simulink model "brake_ctrl"  (R2025b)
settings: Solver=VariableStepAuto  StartTime=0.0  StopTime=10.0  RelTol=1e-3
settings Model: Creator=markk  LastModifiedBy=markk

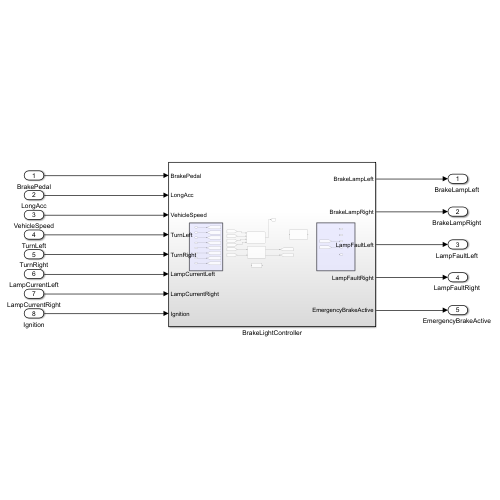
[thumbnail: Simulink's stored preview of the top-level diagram]
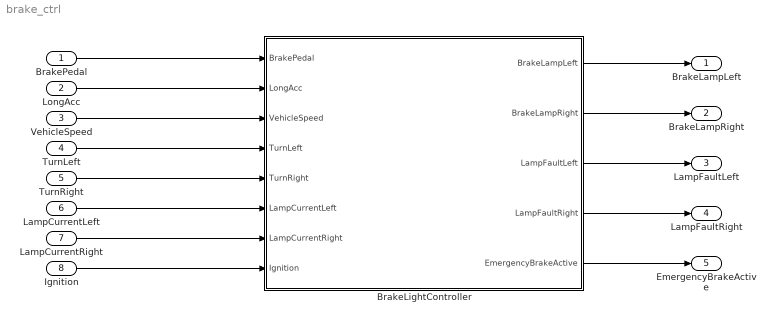
== system brake_ctrl ==
  BrakePedal : Inport
  LongAcc : Inport  Port=2
  VehicleSpeed : Inport  Port=3
  TurnLeft : Inport  Port=4
  TurnRight : Inport  Port=5
  LampCurrentLeft : Inport  Port=6
  LampCurrentRight : Inport  Port=7
  Ignition : Inport  Port=8
  BrakeLightController : Subsystem
  "BrakeLampLeft " : Outport
  "BrakeLampRight " : Outport  Port=2
  "LampFaultLeft " : Outport  Port=3
  "LampFaultRight " : Outport  Port=4
  "EmergencyBrakeActive " : Outport  Port=5
  wires:
  BrakePedal/1 -> BrakeLightController/1(BrakePedal)
  LongAcc/1 -> BrakeLightController/2(LongAcc)
  VehicleSpeed/1 -> BrakeLightController/3(VehicleSpeed)
  TurnLeft/1 -> BrakeLightController/4(TurnLeft)
  TurnRight/1 -> BrakeLightController/5(TurnRight)
  LampCurrentLeft/1 -> BrakeLightController/6(LampCurrentLeft)
  LampCurrentRight/1 -> BrakeLightController/7(LampCurrentRight)
  Ignition/1 -> BrakeLightController/8(Ignition)
  BrakeLightController/1(BrakeLampLeft) -> "BrakeLampLeft "/1
  BrakeLightController/2(BrakeLampRight) -> "BrakeLampRight "/1
  BrakeLightController/3(LampFaultLeft) -> "LampFaultLeft "/1
  BrakeLightController/4(LampFaultRight) -> "LampFaultRight "/1
  BrakeLightController/5(EmergencyBrakeActive) -> "EmergencyBrakeActive "/1

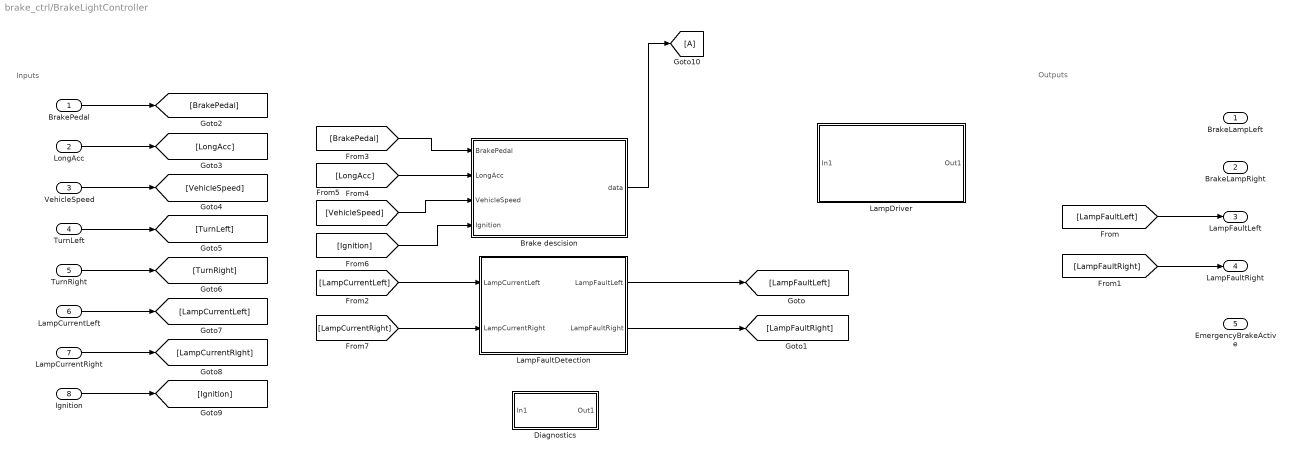
== system brake_ctrl/BrakeLightController ==
  note: Inputs
  note: Outputs
  BrakePedal : Inport
  LongAcc : Inport  Port=2
  VehicleSpeed : Inport  Port=3
  TurnLeft : Inport  Port=4
  TurnRight : Inport  Port=5
  LampCurrentLeft : Inport  Port=6
  LampCurrentRight : Inport  Port=7
  Ignition : Inport  Port=8
  Brake descision : Stateflow chart  TreatAsAtomicUnit=on
  Diagnostics : Subsystem
  Goto10 : Goto
  LampDriver : Subsystem
  LampFaultDetection : Subsystem
  BrakeLampLeft : Outport
  BrakeLampRight : Outport  Port=2
  LampFaultLeft : Outport  Port=3
  LampFaultRight : Outport  Port=4
  EmergencyBrakeActive : Outport  Port=5
  wires:
  Brake descision/1(data) -> Goto10/1
  LampFaultDetection/1(LampFaultLeft) -> [LampFaultLeft]
  LampFaultDetection/2(LampFaultRight) -> [LampFaultRight]
  [LampFaultLeft] -> LampFaultLeft/1
  [LampFaultRight] -> LampFaultRight/1
  BrakePedal/1 -> [BrakePedal]
  LongAcc/1 -> [LongAcc]
  VehicleSpeed/1 -> [VehicleSpeed]
  TurnLeft/1 -> [TurnLeft]
  TurnRight/1 -> [TurnRight]
  LampCurrentLeft/1 -> [LampCurrentLeft]
  LampCurrentRight/1 -> [LampCurrentRight]
  Ignition/1 -> [Ignition]
  [BrakePedal] -> Brake descision/1(BrakePedal)
  [LongAcc] -> Brake descision/2(LongAcc)
  [VehicleSpeed] -> Brake descision/3(VehicleSpeed)
  [Ignition] -> Brake descision/4(Ignition)
  [LampCurrentLeft] -> LampFaultDetection/1(LampCurrentLeft)
  [LampCurrentRight] -> LampFaultDetection/2(LampCurrentRight)

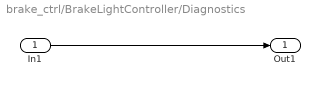
== system brake_ctrl/BrakeLightController/Diagnostics ==
  In1 : Inport
  Out1 : Outport
  wires:
  In1/1 -> Out1/1

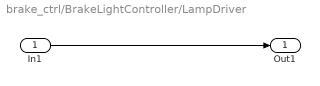
== system brake_ctrl/BrakeLightController/LampDriver ==
  In1 : Inport
  Out1 : Outport
  wires:
  In1/1 -> Out1/1

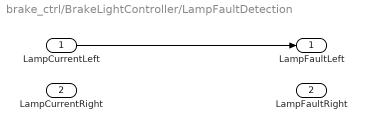
== system brake_ctrl/BrakeLightController/LampFaultDetection ==
  LampCurrentLeft : Inport
  LampCurrentRight : Inport  Port=2
  LampFaultLeft : Outport
  LampFaultRight : Outport  Port=2
  wires:
  LampCurrentLeft/1 -> LampFaultLeft/1

== stateflow chart brake_ctrl/BrakeLightController/Brake descision ==
  state Idle
  state Brake_ON
  state ReleaseHold
  (default) -> Idle
  data: BrakePedal input; LongAcc input; VehicleSpeed input; Ignition input; data output
